simulink model "sedemo_absbrake_can"  (Simulink 7.5)
settings: Solver=ode45  SolverMode=SingleTasking  StartTime=0.0  StopTime=17  MaxStep=inf  RelTol=2e-2  AbsTol=1e-4
PreLoadFcn:
  | sedemo_absdata;
  | BUSCapacity = 50000;
StopFcn:
  | if exist ('logsout')
  | tagName = 'Net';
  | sedemo_absbrakeplots_delay;
  | clear figExt tagName;
  | end
values from neighbouring files (symbols this model uses):
  ctrl = 1    [sedemo_absdata.m]
  g = 32.18    [sedemo_absdata.m]
  I = 5    [sedemo_absdata.m]
  Kf = 1    [sedemo_absdata.m]
  m = 50    [sedemo_absdata.m]
  mu = [0 .4 .8 .97 1.0 .98 .96 .94 .92 .9 .88 .855 .83 .81 .79 .77 .75 .73 .72 .71 .7]    [sedemo_absdata.m]
  PBmax = 1500    [sedemo_absdata.m]
  Rr = 15/12    (= 1.25)    [sedemo_absdata.m]
  slip = (0:.05:1.0)    [sedemo_absdata.m]
  TB = 0.01    [sedemo_absdata.m]
  v0 = 88    [sedemo_absdata.m]
undefined symbols (not defined in the file or in its folder): des_subsystemblock, des_subsysteminport, des_subsystemoutport, des_subsystemsupportblock
libraries: simeventsrouting1 x30, simeventstranslate1 x25, simeventssink1 x21, simeventsserver1 x19, simeventsattributes2 x15, simeventsgates1 x10, simeventsqueue1 x6, simulink x5, simeventsgenerators1 x5, simeventssignalmanage1 x5, simeventstiming1 x3, simeventsinfo x1
(part 1 of 4)
CloseFcn:
  | tagName = 'Net';
  | h = findobj(0, 'Name', 'ABS Speeds', 'Tag', tagName);
  | delete(h);
  | h = findobj(0, 'Name',  'ABS Slip', 'Tag', tagName);
  | delete(h);
  | clear h figExt tagName I PBmax Sd Vs ctrl logsout mu slp v0;
  | clear Kf Rr TB Ww g m slip time BUSCapacity;
  | clear global BUSCapacity;
settings Model: Creator=The MathWorks Inc.  ExtModeTrigMode=oneshot  ExtModeArmWhenConnect=off  ExtModeAutoUpdateStatusClock=off
settings DataIOCC: LimitDataPoints=off  SaveOutput=off  SaveTime=off  TimeSaveName=time
settings OptimizationCC: InlineParams=on  InlineInvariantSignals=on  InitFltsAndDblsToZero=on  EfficientMapNaN2IntZero=off  BufferReusableBoundary=off
settings DebuggingCC: SignalResolutionControl=TryResolveAllWithWarning  SolverPrmCheckMsg=none  MultiTaskDSMMsg=warning  MultiTaskCondExecSysMsg=none  SigSpecEnsureSampleTimeMsg=none  IntegerOverflowMsg=none  BusObjectLabelMismatch=none  StrictBusMsg=None
settings HardwareCC: TargetUnknown=on
settings RTWCC: IncludeERTFirstTime=on
settings SimEventsCC: propMaxDesBlkSimulEvents=10000  propDiagAttribOutput=1  propDiagFcnCallOutput=1  propDiagStatOutput=0

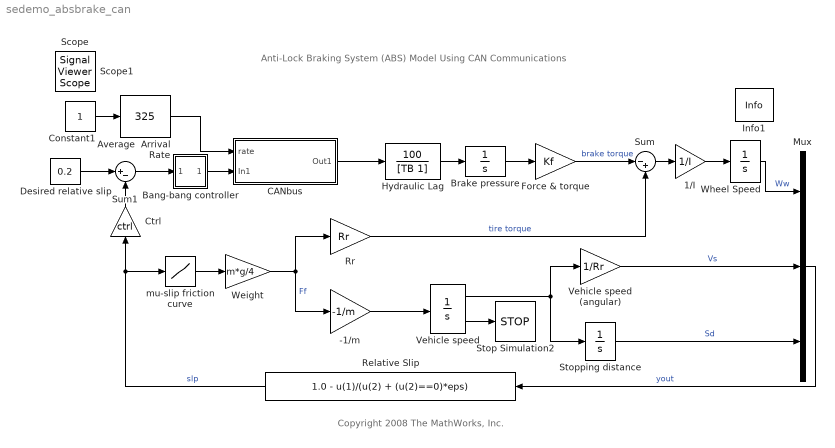
== system sedemo_absbrake_can ==
  note: Anti-Lock Braking System (ABS) Model Using CAN Communications
  note: Copyright 2008 The MathWorks, Inc.
  -1/m : Gain  Gain=-1/m  ParameterDataType=sfix(16)  ParameterScaling=2^0  OutDataType=sfix(16)  OutScaling=2^0  SaturateOnIntegerOverflow=on  OutDataTypeStr=Inherit: Same as input  ParamDataTypeStr=Inherit: Same as input
  1/I : Gain  Gain=1/I  ParameterDataType=sfix(16)  ParameterScaling=2^0  OutDataType=sfix(16)  OutScaling=2^0  SaturateOnIntegerOverflow=on  OutDataTypeStr=Inherit: Same as input  ParamDataTypeStr=Inherit: Same as input
  Average  Arrival Rate : simulink/Math Operations/Slider Gain  SystemSampleTime=-1  low=0  gain=325  high=450
  Bang-bang controller : Subsystem
      mask Type: Sign
      mask Description: y = sign(x)
      mask Help: Sign Function:\n\t\t\ty = 1 if x > 0\n\t\t\ty = 0 if x = 0\n\t\t\ty = -1 if x < 0
      mask Display: plot(-50,-50,50,50,[-50,50],[0,0],[0,0],[-50,50],[-40,0],[-30,-30],[0,40],[30,30])
  Brake pressure : Integrator  LimitOutput=on  UpperSaturationLimit=PBmax  LowerSaturationLimit=0
  CANbus : Subsystem
  Constant1 : Constant  OutDataType=sfix(16)  OutScaling=2^0
  Ctrl : Gain  Gain=ctrl  ParameterDataType=sfix(16)  ParameterScaling=2^0  OutDataType=sfix(16)  OutScaling=2^0  SaturateOnIntegerOverflow=on  OutDataTypeStr=Inherit: Same as input  ParamDataTypeStr=Inherit: Same as input
  Desired relative slip : Constant  Value=0.2  OutDataType=sfix(16)  OutScaling=2^0
  Force & torque : Gain  Gain=Kf  ParameterDataType=sfix(16)  ParameterScaling=2^0  OutDataType=sfix(16)  OutScaling=2^0  SaturateOnIntegerOverflow=on  OutDataTypeStr=Inherit: Same as input  ParamDataTypeStr=Inherit: Same as input
  "Hydraulic Lag " : TransferFcn  Numerator=[100]  Denominator=[TB 1]
  Info1 : simeventsinfo/Info  SystemSampleTime=-1
  Mux : Mux  Inputs=3
  Relative Slip : Fcn  Expr=1.0 - u(1)/(u(2) + (u(2)==0)*eps)
  Rr : Gain  Gain=Rr  ParameterDataType=sfix(16)  ParameterScaling=2^0  OutDataType=sfix(16)  OutScaling=2^0  SaturateOnIntegerOverflow=on  OutDataTypeStr=Inherit: Same as input  ParamDataTypeStr=Inherit: Same as input
  Stop Simulation2 : Stop
  Stopping distance : Integrator  UpperSaturationLimit=1000  LowerSaturationLimit=0
  Sum : Sum  Inputs=|-+  OutDataType=sfix(16)  OutScaling=2^0  SaturateOnIntegerOverflow=on  InputSameDT=on  OutDataTypeStr=Inherit: Same as first input
  Sum1 : Sum  Inputs=|+-  OutDataType=sfix(16)  OutScaling=2^0  SaturateOnIntegerOverflow=on  InputSameDT=on  OutDataTypeStr=Inherit: Same as first input
  Vehicle speed : Integrator  InitialCondition=v0  LimitOutput=on  UpperSaturationLimit=1000  LowerSaturationLimit=0  ShowSaturationPort=on
  Vehicle speed (angular) : Gain  Gain=1/Rr  ParameterDataType=sfix(16)  ParameterScaling=2^0  OutDataType=sfix(16)  OutScaling=2^0  SaturateOnIntegerOverflow=on  OutDataTypeStr=Inherit: Same as input  ParamDataTypeStr=Inherit: Same as input
  Weight : Gain  Gain=m*g/4  ParameterDataType=sfix(16)  ParameterScaling=2^0  OutDataType=sfix(16)  OutScaling=2^0  SaturateOnIntegerOverflow=on  OutDataTypeStr=Inherit: Same as input  ParamDataTypeStr=Inherit: Same as input
  Wheel Speed : Integrator  InitialCondition=v0/Rr  LimitOutput=on  UpperSaturationLimit=1000  LowerSaturationLimit=0
  mu-slip friction curve : Lookup  InputValues=slip  Table=mu  OutDataType=sfix(16)  OutScaling=2^0  SaturateOnIntegerOverflow=on
  Scope : SignalViewerScope  IOType=viewer  RefreshTime=0.035000
      settings: TimeRange=15  YMin=0  YMax=800
  Scope1 : SignalViewerScope  IOType=viewer  RefreshTime=0.035000
      settings: TimeRange=15  YMin=0  YMax=1
  wires:
  Mux/1 -> Relative Slip/1  "yout"
  Vehicle speed (angular)/1 -> Mux/2  "Vs"
  Relative Slip/1 -> mu-slip friction curve/1, Ctrl/1  "slp"
  Stopping distance/1 -> Mux/3  "Sd"
  -1/m/1 -> Vehicle speed/1
  Vehicle speed/2 -> Stop Simulation2/1
  Vehicle speed/1 -> Stopping distance/1, Vehicle speed (angular)/1
  mu-slip friction curve/1 -> Weight/1
  Weight/1 -> -1/m/1, Rr/1  "Ff"
  Ctrl/1 -> Sum1/2
  Desired relative slip/1 -> Sum1/1
  Sum1/1 -> Bang-bang controller/1(in_1)
  Wheel Speed/1 -> Mux/1  "Ww"
  Rr/1 -> Sum/2  "tire torque"
  1/I/1 -> Wheel Speed/1
  Sum/1 -> 1/I/1
  Force & torque/1 -> Sum/1  "brake torque"
  Brake pressure/1 -> Force & torque/1
  "Hydraulic Lag "/1 -> Brake pressure/1
  Constant1/1 -> Average  Arrival Rate/1
  Average  Arrival Rate/1 -> CANbus/1(rate)
  Bang-bang controller/1(out_1) -> CANbus/2(In1)
  CANbus/1(Out1) -> "Hydraulic Lag "/1

== system sedemo_absbrake_can/Bang-bang controller ==
  in_1 : Inport  OutDataType=sfix(16)  OutScaling=2^0
  Constant : Constant  Value=0  OutDataType=sfix(16)  OutScaling=2^0
  Data Type Conversion1 : DataTypeConversion  OutDataTypeMode=double  OutDataType=sfix(16)  OutScaling=2^0  OutDataTypeStr=double  SaturateOnIntegerOverflow=on  RndMeth=Zero
  Data Type Conversion2 : DataTypeConversion  OutDataTypeMode=double  OutDataType=sfix(16)  OutScaling=2^0  OutDataTypeStr=double  SaturateOnIntegerOverflow=on  RndMeth=Zero
  Relational Operator : RelationalOperator  Operator=>  InputSameDT=on
  Relational Operator1 : RelationalOperator  Operator=<  InputSameDT=on
  Sum : Sum  Inputs=+-  OutDataType=sfix(16)  OutScaling=2^0  SaturateOnIntegerOverflow=on  InputSameDT=on  OutDataTypeStr=Inherit: Same as first input
  out_1 : Outport  OutDataType=sfix(16)  OutScaling=2^0  InitialOutput=0
  wires:
  Data Type Conversion2/1 -> Sum/2
  Data Type Conversion1/1 -> Sum/1
  Sum/1 -> out_1/1
  Relational Operator/1 -> Data Type Conversion1/1
  Relational Operator1/1 -> Data Type Conversion2/1
  Constant/1 -> Relational Operator/2, Relational Operator1/2
  in_1/1 -> Relational Operator1/1, Relational Operator/1

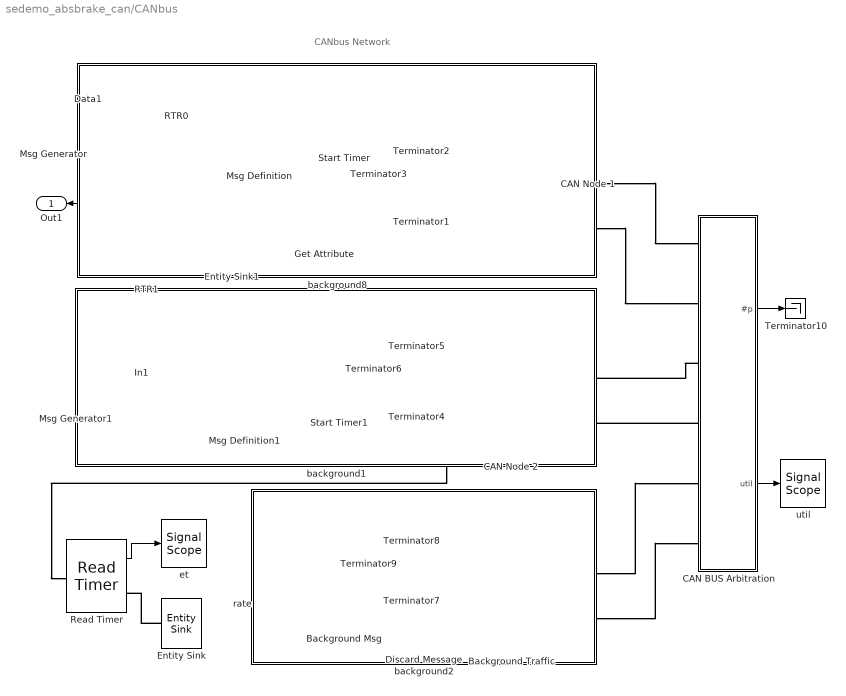
== system sedemo_absbrake_can/CANbus ==
  note: CANbus Network
  rate : Inport  OutDataType=sfix(16)  OutScaling=2^0
  In1 : Inport  Port=2  OutDataType=sfix(16)  OutScaling=2^0
  Background Msg : Subsystem
  Background Traffic : Subsystem  mask(Background Traffic){IDRange=[0:9], IDSubscription=[zeros(1,10)]}
      mask prompts: IDRange "Message ID"; IDSubscription "Subscription (0-no, 1-yes)"
      mask help: Transmits and receives messages to and from multiple nodes over the CANbus to represent background traffic on the CANbus.
  CAN BUS Arbitration : Subsystem  mask{Capacity=50000, LossRate=0.001}
      mask prompts: Capacity "Channel capacity(bit/s)"; LossRate "Loss probability(0-1)"
      mask init:
      | global BUSCapacity;
      | BUSCapacity = Capacity;
  CAN Node 1 : Subsystem  mask(CAN Node){IDRange=[0:9], IDSubscription=[0,0,0,1,0,0,0,0,0,0]}
      mask prompts: IDRange "Message ID"; IDSubscription "Subscription (0-no, 1-yes)"
      mask help: CAN Node transmits and receives messages over the CANbus.
  CAN Node 2 : Subsystem  mask(CAN Node){IDRange=[0:9], IDSubscription=[0,0,1,0,0,0,0,0,0,0]}
      mask prompts: IDRange "Message ID"; IDSubscription "Subscription (0-no, 1-yes)"
      mask help: CAN Node transmits and receives messages over the CANbus.
  Data1 : simulink/Sources/Ramp  SystemSampleTime=-1  slope=1  start=0  X0=0
  Discard Message : simeventssink1/Entity Sink  Priority=1  SystemSampleTime=-1  AvailableForArrivals=on  StatNumberArrived=Off
  Entity Sink : simeventssink1/Entity Sink  Priority=1  SystemSampleTime=-1  AvailableForArrivals=on  StatNumberArrived=Off
  Entity Sink1 : simeventssink1/Entity Sink  Priority=1  SystemSampleTime=-1  AvailableForArrivals=on  StatNumberArrived=Off
  Get Attribute : simeventsattributes2/Get Attribute  Priority=1  DialogController=des_ddg_create  DialogControllerArgs=DataTag206  SystemSampleTime=-1  AttributeName=Data  AttributeMissing=Error  AttributeDefaultValue=1  AttributeSendTiming=After entity departure  AttributeTreatAsVector=1  StatNumberDeparted=Off  EvaluatedDefaultAttributeValue={[]}
  Msg Definition : Subsystem  mask{MsgID=2, MsgSize=8}
      mask prompts: MsgID "CAN identifier (ID)"; MsgSize "Data size (0-8 bytes)"
      settings: AttributesFormatString=(ID = %<MsgID>)
  Msg Definition1 : Subsystem  mask{MsgID=3, MsgSize=8}
      mask prompts: MsgID "CAN identifier (ID)"; MsgSize "Data size (0-8 bytes)"
      settings: AttributesFormatString=(ID = %<MsgID>)
  Msg Generator : simeventsgenerators1/Entity Generators/Time-Based Entity Generator  Priority=1  DialogController=des_ddg_create  DialogControllerArgs=DataTag212  SystemSampleTime=-1  GenerateEntitiesUpon=Intergeneration time from dialog  Distribution=Constant  Minimum=0  Maximum=1  Mean=0.05  InitialSeed=568654  Period=0.333  PriorityEntityGeneration=300  GenerateEntityAtSimulationStart=off  ResponseWhenBlocked=Pause generation  ResponseWhenUnblocked=Immediate restart  EntityType=Standard  StatNumberDeparted=Off  StatPendingEntity=Off  StatAverageIntergenerationTime=Off
  Msg Generator1 : simeventsgenerators1/Entity Generators/Time-Based Entity Generator  Priority=1  DialogController=des_ddg_create  DialogControllerArgs=DataTag214  SystemSampleTime=-1  GenerateEntitiesUpon=Intergeneration time from dialog  Distribution=Constant  Minimum=0  Maximum=1  Mean=0.05  InitialSeed=5363461  Period=0.01  PriorityEntityGeneration=300  GenerateEntityAtSimulationStart=off  ResponseWhenBlocked=Pause generation  ResponseWhenUnblocked=Immediate restart  EntityType=Standard  StatNumberDeparted=Off  StatPendingEntity=Off  StatAverageIntergenerationTime=Off
  RTR0 : Constant  Value=0  OutDataType=sfix(16)  OutScaling=2^0
  RTR1 : Constant  Value=0  OutDataType=sfix(16)  OutScaling=2^0
  Read Timer : simeventstiming1/Read Timer  Priority=0  SystemSampleTime=-1  TimerTag=T1  TimerModeOption=Error  TimerStop=off  StatNumberDeparted=Off  StatTimerNumberDeparted=Off  StatTimeElapsed=On  StatAverageTimeElapsed=Off
  Start Timer : simeventstiming1/Start Timer  Priority=0  SystemSampleTime=-1  TimerTag=T1  TimerStartedOption=Warn and continue  StatNumberDeparted=Off
  Start Timer1 : simeventstiming1/Start Timer  Priority=0  SystemSampleTime=-1  TimerTag=T1  TimerStartedOption=Warn and continue  StatNumberDeparted=Off
  Terminator{1..10} (10 alike) : Terminator
  background1 : Subsystem
      mask Display: disp('')
  background2 : Subsystem
      mask Display: disp('')
  background8 : Subsystem
      mask Display: disp('')
  et : simeventssink1/Signal Scope  Priority=1  SystemSampleTime=-1  PlotType=Stair  InputType=Signal  NumInputs=1  AttributeNameY=Count  XInputOptionSignal=Event time  XInputOptionEntity=Event time  AttributeNameX=Count  EnableEntityOutport=on  XMin=0  XMax=18  XLimitExceededOption=Stretch axis limits  YLimitExceededOption=Stretch axis limits  AxisGrid=on  AxisLegend=off  LineDisables=""  LineColors=b  LineStyles=-  LineMarkers=None  OpenScopeAtSimStart=on  Title=Message Delivery Delay  YLabel=Delay  XLabel=Time  FigurePosition=[461 438 307 230]  AxisZoom=off  DataStoreOption=Unlimited  DataPointsLimit=10000  StatNumberArrived=Off  ShowCountPlotted=off  ShowToolbar=off
      settings: YMin=0  YMax=0.005
  util : simeventssink1/Signal Scope  Priority=1  SystemSampleTime=-1  PlotType=Stair  InputType=Signal  NumInputs=1  AttributeNameY=Count  XInputOptionSignal=Event time  XInputOptionEntity=Event time  AttributeNameX=Count  EnableEntityOutport=on  XMin=0  XMax=18  XLimitExceededOption=Stretch axis limits  YLimitExceededOption=Stretch axis limits  AxisGrid=on  AxisLegend=off  LineDisables=""  LineColors=b  LineStyles=-  LineMarkers=None  OpenScopeAtSimStart=on  Title=CANbus Network Utilization  YLabel=Utilization  XLabel=Time  FigurePosition=[51 437 307 230]  AxisZoom=off  DataStoreOption=Unlimited  DataPointsLimit=10000  StatNumberArrived=Off  ShowCountPlotted=off  ShowToolbar=off
      settings: YMin=0  YMax=1
  Out1 : Outport  OutDataType=sfix(16)  OutScaling=2^0
  wires:
  Get Attribute/1 -> Out1/1
  rate/1 -> Background Msg/1(rate)
  CAN BUS Arbitration/1(#p) -> Terminator10/1
  CAN BUS Arbitration/2(util) -> util/1
  Background Traffic/4(#Tx) -> Terminator7/1
  Background Traffic/3(#OF) -> Terminator9/1
  Background Traffic/1(#Rx) -> Terminator8/1
  Background Traffic/2(#Bx) -> Background Traffic/1(Idx)
  Read Timer/1 -> et/1
  CAN Node 2/4(#Tx) -> Terminator4/1
  CAN Node 2/3(#OF) -> Terminator6/1
  CAN Node 2/1(#Rx) -> Terminator5/1
  RTR1/1 -> Msg Definition1/1(RTR)
  In1/1 -> Msg Definition1/2(Data)
  CAN Node 2/2(#Bx) -> CAN Node 2/1(Idx)
  CAN Node 1/4(#Tx) -> Terminator1/1
  CAN Node 1/3(#OF) -> Terminator3/1
  CAN Node 1/1(#Rx) -> Terminator2/1
  RTR0/1 -> Msg Definition/1(RTR)
  Data1/1 -> Msg Definition/2(Data)
  CAN Node 1/2(#Bx) -> CAN Node 1/1(Idx)
  connections:
  Entity Sink1/LConn1 -- Get Attribute/RConn1
  Get Attribute/LConn1 -- CAN Node 1/RConn2
  Background Msg/RConn1 -- Background Traffic/RConn1
  CAN Node 1/LConn2 -- CAN BUS Arbitration/LConn2
  CAN Node 1/LConn1 -- CAN BUS Arbitration/LConn1
  Entity Sink/LConn1 -- Read Timer/RConn1
  Msg Generator/RConn1 -- Msg Definition/LConn1
  Start Timer1/RConn1 -- CAN Node 2/RConn1
  Background Traffic/LConn2 -- CAN BUS Arbitration/LConn6
  Msg Definition/RConn1 -- Start Timer/LConn1
  Msg Generator1/RConn1 -- Msg Definition1/LConn1
  Msg Definition1/RConn1 -- Start Timer1/LConn1
  Start Timer/RConn1 -- CAN Node 1/RConn1
  CAN BUS Arbitration/LConn3 -- CAN Node 2/LConn1
  Background Traffic/LConn1 -- CAN BUS Arbitration/LConn5
  CAN Node 2/RConn2 -- Read Timer/LConn1
  CAN BUS Arbitration/LConn4 -- CAN Node 2/LConn2
  Discard Message/LConn1 -- Background Traffic/RConn2

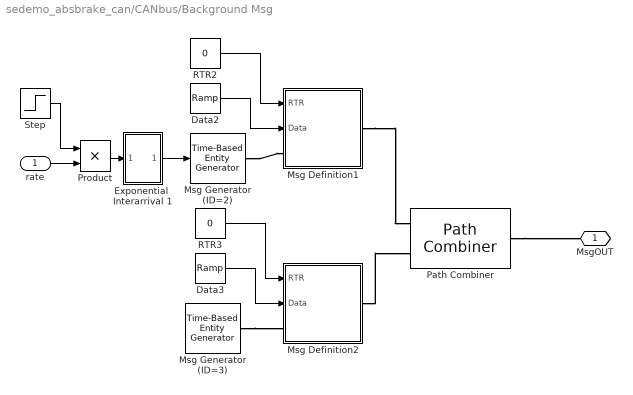
== system sedemo_absbrake_can/CANbus/Background Msg ==
  rate : Inport  OutDataType=sfix(16)  OutScaling=2^0
  Data2 : simulink/Sources/Ramp  SystemSampleTime=-1  slope=1  start=0  X0=0
  Data3 : simulink/Sources/Ramp  SystemSampleTime=-1  slope=1  start=0  X0=0
  Exponential  Interarrival 1 : Subsystem  mask(Exponential Random Number Generator){seed=0546269209}
      mask prompts: seed "Initial seed"
      mask help: Generate random numbers with an exponential distribution. User can specify the rate and the initial seed.
      mask Display: plot([0.4 .13 .38 .26 .71 .44 .6 .15 .22 .5 .55 .6 .4]);
  Msg Definition1 : Subsystem  mask{MsgID=0, MsgSize=8}
      mask prompts: MsgID "CAN identifier (ID)"; MsgSize "Data size (0-8 bytes)"
      settings: AttributesFormatString=(ID = %<MsgID>)
  Msg Definition2 : Subsystem  mask{MsgID=1, MsgSize=8}
      mask prompts: MsgID "CAN identifier (ID)"; MsgSize "Data size (0-8 bytes)"
      settings: AttributesFormatString=(ID = %<MsgID>)
  Msg Generator (ID=2) : simeventsgenerators1/Entity Generators/Time-Based Entity Generator  Priority=1  DialogController=des_ddg_create  DialogControllerArgs=DataTag5  SystemSampleTime=-1  GenerateEntitiesUpon=Intergeneration time from port t  Distribution=Exponential  Minimum=0  Maximum=1  Mean=0.02  InitialSeed=67457  Period=0.05  PriorityEntityGeneration=300  GenerateEntityAtSimulationStart=off  ResponseWhenBlocked=Pause generation  ResponseWhenUnblocked=Immediate restart  EntityType=Standard  StatNumberDeparted=Off  StatPendingEntity=Off  StatAverageIntergenerationTime=Off
  Msg Generator (ID=3) : simeventsgenerators1/Entity Generators/Time-Based Entity Generator  Priority=1  DialogController=des_ddg_create  DialogControllerArgs=DataTag7  SystemSampleTime=-1  GenerateEntitiesUpon=Intergeneration time from dialog  Distribution=Constant  Minimum=.04  Maximum=.1  Mean=0.08  InitialSeed=3767  Period=inf  PriorityEntityGeneration=300  GenerateEntityAtSimulationStart=off  ResponseWhenBlocked=Pause generation  ResponseWhenUnblocked=Immediate restart  EntityType=Standard  StatNumberDeparted=Off  StatPendingEntity=Off  StatAverageIntergenerationTime=Off
  Path Combiner : simeventsrouting1/Path Combiner  Priority=1  SystemSampleTime=-1  NumberInputPorts=2  InputPortPrecedence=IN1 port  InitialSeed=45675  SpecifyEventPriority=off  PriorityPathCombinerPortPrecedenceSelection=4100  StatNumberDeparted=Off  StatLastArrivalPort=Off  EvaluatedNumPorts=2
  Product : Product  OutDataType=sfix(16)  OutScaling=2^0  RndMeth=Zero
  RTR2 : Constant  Value=0  OutDataType=sfix(16)  OutScaling=2^0
  RTR3 : Constant  Value=0  OutDataType=sfix(16)  OutScaling=2^0
  Step : Step  Time=6  Before=.01  SampleTime=0
  MsgOUT : PMIOPort  Port=1  Side=Right
  wires:
  rate/1 -> Product/2
  Product/1 -> Exponential  Interarrival 1/1(rate)
  Step/1 -> Product/1
  Exponential  Interarrival 1/1(Out1) -> Msg Generator (ID=2)/1
  RTR3/1 -> Msg Definition2/1(RTR)
  Data3/1 -> Msg Definition2/2(Data)
  RTR2/1 -> Msg Definition1/1(RTR)
  Data2/1 -> Msg Definition1/2(Data)
  connections:
  Msg Definition1/RConn1 -- Path Combiner/LConn1
  Msg Definition2/RConn1 -- Path Combiner/LConn2
  Path Combiner/RConn1 -- MsgOUT/RConn1
  Msg Generator (ID=3)/RConn1 -- Msg Definition2/LConn1
  Msg Generator (ID=2)/RConn1 -- Msg Definition1/LConn1

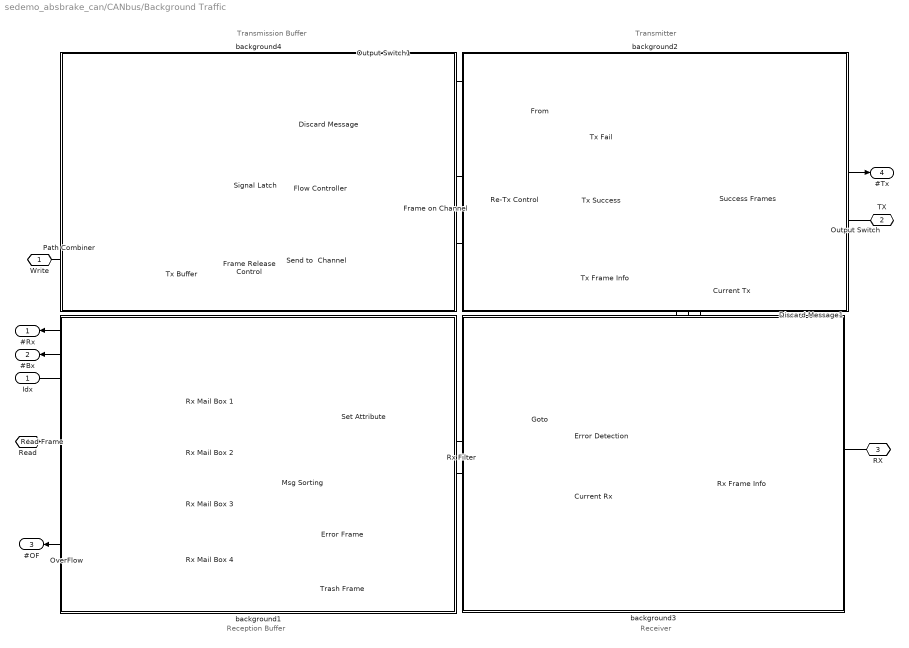
== system sedemo_absbrake_can/CANbus/Background Traffic ==
  note: Reception Buffer
  note: Transmission Buffer
  note: Transmitter
  note: Receiver
  Idx : Inport  OutDataType=sfix(16)  OutScaling=2^0
  Current Rx : simeventsserver1/Single Server  Priority=1  SystemSampleTime=-1  ServiceTimeFrom=Dialog  ServiceTime=0  AttributeName=ServiceTime  PriorityServiceCompletion=2400  PermitPreemption=off  SortingAttributeName=ID  SortingDirection=Ascending  WriteToAttribute=off  ResidualAttributeName=ResidualServiceTime  CreateAttribute=on  EnableTOPort=off  StatNumberDeparted=Off  StatNumberInBlock=Off  StatNumberPreempted=Off  StatPendingEntity=Off  StatAverageWait=Off  StatUtilization=Off  StatNumberTimedout=Off
  Current Tx : simeventsserver1/Single Server  Priority=1  SystemSampleTime=-1  ServiceTimeFrom=Dialog  ServiceTime=0  AttributeName=ServiceTime  PriorityServiceCompletion=2400  PermitPreemption=off  SortingAttributeName=ID  SortingDirection=Ascending  WriteToAttribute=off  ResidualAttributeName=ResidualServiceTime  CreateAttribute=on  EnableTOPort=off  StatNumberDeparted=Off  StatNumberInBlock=Off  StatNumberPreempted=Off  StatPendingEntity=Off  StatAverageWait=Off  StatUtilization=Off  StatNumberTimedout=Off
  Discard Message : simeventssink1/Entity Sink  Priority=1  SystemSampleTime=-1  AvailableForArrivals=on  StatNumberArrived=Off
  Discard Message1 : simeventssink1/Entity Sink  Priority=1  SystemSampleTime=-1  AvailableForArrivals=on  StatNumberArrived=Off
  Error Detection : Subsystem  LoadFcn=des_subsystemblock(gcb, 'load');  InitFcn=des_subsystemblock(gcb, 'init');  StartFcn=des_subsystemblock(gcb, 'start');  StopFcn=des_subsystemblock(gcb, 'stop');
      settings: CopyFcn=des_subsystemblock(gcb, 'copy');  DeleteFcn=des_subsystemblock(gcb, 'delete');  UndoDeleteFcn=des_subsystemblock(gcb, 'undodelete');  ModelCloseFcn=des_subsystemblock(gcb, 'modelclose');  PreSaveFcn=des_subsystemblock(gcb, 'presave');  NameChangeFcn=des_subsystemblock(gcb, 'namechange');  ParentCloseFcn=des_subsystemblock(gcb, 'parentclose');  ErrorFcn=des_subsystemerror
  Error Frame : simeventssink1/Entity Sink  Priority=1  SystemSampleTime=-1  AvailableForArrivals=on  StatNumberArrived=Off
  Flow Controller : Subsystem  LoadFcn=des_subsystemblock(gcb, 'load');  InitFcn=des_subsystemblock(gcb, 'init');  StartFcn=des_subsystemblock(gcb, 'start');  StopFcn=des_subsystemblock(gcb, 'stop');
      settings: CopyFcn=des_subsystemblock(gcb, 'copy');  DeleteFcn=des_subsystemblock(gcb, 'delete');  UndoDeleteFcn=des_subsystemblock(gcb, 'undodelete');  ModelCloseFcn=des_subsystemblock(gcb, 'modelclose');  PreSaveFcn=des_subsystemblock(gcb, 'presave');  NameChangeFcn=des_subsystemblock(gcb, 'namechange');  ParentCloseFcn=des_subsystemblock(gcb, 'parentclose');  ErrorFcn=des_subsystemerror
  Frame Release Control : simeventsgates1/Enabled Gate  Priority=1  SystemSampleTime=-1  SpecifyEventPriority=on  PriorityGateEnableOpenClose=2300  StatNumberDeparted=Off
  Frame on Channel : simeventsqueue1/FIFO Queue  Priority=1  SystemSampleTime=-1  Capacity=2  EnableTOPort=off  StatNumberDeparted=Off  StatNumberInBlock=On  StatPendingEntity=Off  StatAverageWait=Off  StatAverageQueueLength=Off  StatNumberTimedout=Off
  Msg Sorting : simeventsrouting1/Output Switch  Priority=1  SystemSampleTime=-1  NumberOutputPorts=4  SwitchingCriterion=Round robin  InitialSeed=34567  AttributeName=Attribute1  InitialConditionsOpt=off  InitialConditions=1  EntityBufferOpt=off  SpecifyEventPriority=off  PriorityOutputSwitchSelectPort=4100  TimeoutPortOpt=off  StatNumberDeparted=On  StatNumberTimedOut=Off  StatPendingEntity=Off  StatLastDeparturePort=On  EvaluatedNumPorts=4
  Output Switch : simeventsrouting1/Output Switch  Priority=1  SystemSampleTime=-1  NumberOutputPorts=2  SwitchingCriterion=First port that is not blocked  InitialSeed=34567  AttributeName=Attribute1  InitialConditionsOpt=off  InitialConditions=1  EntityBufferOpt=off  SpecifyEventPriority=off  PriorityOutputSwitchSelectPort=4100  TimeoutPortOpt=off  StatNumberDeparted=Off  StatNumberTimedOut=Off  StatPendingEntity=Off  StatLastDeparturePort=Off  EvaluatedNumPorts=2
  Output Switch1 : simeventsrouting1/Output Switch  Priority=1  SystemSampleTime=-1  NumberOutputPorts=2  SwitchingCriterion=First port that is not blocked  InitialSeed=34567  AttributeName=Attribute1  InitialConditionsOpt=off  InitialConditions=1  EntityBufferOpt=off  SpecifyEventPriority=off  PriorityOutputSwitchSelectPort=4100  TimeoutPortOpt=off  StatNumberDeparted=Off  StatNumberTimedOut=Off  StatPendingEntity=Off  StatLastDeparturePort=Off  EvaluatedNumPorts=2
  OverFlow : simeventsrouting1/Path Combiner  Priority=1  SystemSampleTime=-1  NumberInputPorts=4  InputPortPrecedence=IN1 port  InitialSeed=45675  SpecifyEventPriority=off  PriorityPathCombinerPortPrecedenceSelection=4100  StatNumberDeparted=On  StatLastArrivalPort=Off  EvaluatedNumPorts=4
  Path Combiner : simeventsrouting1/Path Combiner  Priority=1  SystemSampleTime=-1  NumberInputPorts=2  InputPortPrecedence=IN1 port  InitialSeed=45675  SpecifyEventPriority=off  PriorityPathCombinerPortPrecedenceSelection=4100  StatNumberDeparted=Off  StatLastArrivalPort=Off  EvaluatedNumPorts=2
  Re-Tx Control : simeventsrouting1/Output Switch  Priority=1  SystemSampleTime=-1  NumberOutputPorts=2  SwitchingCriterion=First port that is not blocked  InitialSeed=34567  AttributeName=Attribute1  InitialConditionsOpt=off  InitialConditions=1  EntityBufferOpt=off  SpecifyEventPriority=off  PriorityOutputSwitchSelectPort=4100  TimeoutPortOpt=off  StatNumberDeparted=Off  StatNumberTimedOut=Off  StatPendingEntity=Off  StatLastDeparturePort=Off  EvaluatedNumPorts=2
  Read Frame : simeventsrouting1/Input Switch  Priority=1  SystemSampleTime=-1  NumberInputPorts=4  SwitchingCriterion=From signal port p  InitialSeed=23453  SpecifyEventPriority=off  PriorityInputSwitchSelectPort=4000  StatNumberDeparted=Off  StatLastArrivalPort=Off  EvaluatedNumPorts=4
  Rx Filter : simeventsrouting1/Output Switch  Priority=1  SystemSampleTime=-1  NumberOutputPorts=3  SwitchingCriterion=From signal port p  InitialSeed=34567  AttributeName=Attribute1  InitialConditionsOpt=off  InitialConditions=1  EntityBufferOpt=off  SpecifyEventPriority=off  PriorityOutputSwitchSelectPort=4100  TimeoutPortOpt=off  StatNumberDeparted=On  StatNumberTimedOut=Off  StatPendingEntity=Off  StatLastDeparturePort=Off  EvaluatedNumPorts=3
  Rx Frame Info : simeventsattributes2/Get Attribute  Priority=1  DialogController=des_ddg_create  DialogControllerArgs=DataTag52  SystemSampleTime=-1  AttributeName=ID|RndLoss|RTR|Data  AttributeMissing=Error|Error|Error|Error  AttributeDefaultValue=1|1|1|1  AttributeSendTiming=After entity departure|After entity departure|After entity departure|After entity departure  AttributeTreatAsVector=1|1|1|1  StatNumberDeparted=Off  EvaluatedDefaultAttributeValue={[];[];[];[]}
  Rx Mail Box {1..4} (4 alike) : simeventsserver1/Single Server  Priority=1  SystemSampleTime=-1  ServiceTimeFrom=Dialog  ServiceTime=0  AttributeName=ServiceTime  PriorityServiceCompletion=2400  PermitPreemption=on  SortingAttributeName=time  SortingDirection=Descending  WriteToAttribute=off  ResidualAttributeName=ResidualServiceTime  CreateAttribute=on  EnableTOPort=off  StatNumberDeparted=Off  StatNumberInBlock=Off  StatNumberPreempted=Off  StatPendingEntity=Off  StatAverageWait=Off  StatUtilization=Off  StatNumberTimedout=Off
  Send to  Channel : simeventsrouting1/Replicate  Priority=1  SystemSampleTime=-1  NumberOutputPorts=2  ReplicateEntityWhen=All entity output ports are not blocked  OutputPortPrecedence=OUT1 port  InitialSeed=56789  ActionUponBlocking=Discard entity  StatNumberArrived=Off  StatNumberDeparted=Off  EvaluatedNumPorts=2
  Set Attribute : simeventsattributes2/Set Attribute  Priority=1  DialogController=des_ddg_create  DialogControllerArgs=DataTag59  SystemSampleTime=-1  AttributeFrom=Signal port  AttributeName=time  AttributeTreatAsVector=1  AttributeValue=1  AttributeCreate=on  StatNumberDeparted=Off  EvaluatedAttributeValue={[]}
  Signal Latch : simeventssignalmanage1/Signal Latch  Priority=1  SystemSampleTime=-1  InitialMemoryValue=1  WriteMemoryUpon=Sample time hit from port wts  MemoryWriteEdgeOption=Either  SpecifyWriteEventPriority=on  PriorityMemoryWrite=2200  ReadMemoryUpon=Write to memory event  MemoryReadEdgeOption=Falling  SpecifyReadEventPriority=on  PriorityMemoryRead=7000  ReportMemoryState=off  ReportMemoryUponWrite=off  ReportMemoryUponRead=on
  Success Frames : simeventssink1/Entity Sink  Priority=1  SystemSampleTime=-1  AvailableForArrivals=on  StatNumberArrived=On
  Trash Frame : simeventssink1/Entity Sink  Priority=1  SystemSampleTime=-1  AvailableForArrivals=on  StatNumberArrived=Off
  Tx Buffer : simeventsqueue1/Priority Queue  Priority=1  SystemSampleTime=-1  Capacity=15  SortingAttributeName=ID  SortingDirection=Ascending  EnableTOPort=off  StatNumberDeparted=Off  StatNumberInBlock=Off  StatPendingEntity=Off  StatAverageWait=Off  StatAverageQueueLength=Off  StatNumberTimedout=Off
  Tx Fail : simeventsgates1/Release Gate  Priority=1  SystemSampleTime=-1  OpenGateUpon=Change in signal from port vc  SignalEdgeOption=Falling  SpecifyEventPriority=on  PriorityGateRelease=2000  StatNumberDeparted=Off
  Tx Frame Info : simeventsattributes2/Get Attribute  Priority=1  DialogController=des_ddg_create  DialogControllerArgs=DataTag66  SystemSampleTime=-1  AttributeName=ID|RTR|Data  AttributeMissing=Error|Error|Error  AttributeDefaultValue=1|1|1  AttributeSendTiming=After entity departure|After entity departure|After entity departure  AttributeTreatAsVector=1|1|1  StatNumberDeparted=Off  EvaluatedDefaultAttributeValue={[];[];[]}
  Tx Success : simeventsgates1/Release Gate  Priority=1  SystemSampleTime=-1  OpenGateUpon=Change in signal from port vc  SignalEdgeOption=Rising  SpecifyEventPriority=on  PriorityGateRelease=2000  StatNumberDeparted=Off
  background1 : Subsystem
      mask Display: disp('')
  background2 : Subsystem
      mask Display: disp('')
  background3 : Subsystem
      mask Display: disp('')
  background4 : Subsystem
      mask Display: disp('')
  Write : PMIOPort  Port=1  Side=Right
  TX : PMIOPort  Port=2  Side=Left
  RX : PMIOPort  Port=3  Side=Left
  Read : PMIOPort  Port=4  Side=Right
  #Rx : Outport  OutDataType=sfix(16)  OutScaling=2^0
  #Bx : Outport  Port=2  OutDataType=sfix(16)  OutScaling=2^0
  #OF : Outport  Port=3  OutDataType=sfix(16)  OutScaling=2^0
  #Tx : Outport  Port=4  OutDataType=sfix(16)  OutScaling=2^0
  wires:
  Success Frames/1 -> #Tx/1
  Msg Sorting/1 -> #Rx/1
  OverFlow/1 -> #OF/1
  Msg Sorting/2 -> #Bx/1
  Idx/1 -> Read Frame/1
  Signal Latch/1 -> Frame Release Control/1
  Frame on Channel/1 -> Flow Controller/1(busy)
  Rx Filter/1 -> Set Attribute/1
  Rx Frame Info/1 -> Error Detection/1(Rx_ID)
  Rx Frame Info/2 -> Error Detection/2(Loss)
  Tx Frame Info/3 -> Error Detection/7(Tx_Data)
  Tx Frame Info/2 -> Error Detection/6(Tx_RTR)
  Tx Frame Info/1 -> Error Detection/5(Tx_ID)
  Rx Frame Info/3 -> Error Detection/3(Rx_RTR)
  Rx Frame Info/4 -> Error Detection/4(Rx_Data)
  Error Detection/1(Idx) -> Rx Filter/1
  Error Detection/2(ACK) -> [Ack]
  [Ack] -> Tx Fail/1, Tx Success/1
  Flow Controller/1(en) -> Signal Latch/1, Signal Latch/2
  connections:
  Read Frame/RConn1 -- Read/RConn1
  Msg Sorting/RConn4 -- Rx Mail Box 4/LConn1
  Msg Sorting/RConn3 -- Rx Mail Box 3/LConn1
  Msg Sorting/RConn2 -- Rx Mail Box 2/LConn1
  Msg Sorting/RConn1 -- Rx Mail Box 1/LConn1
  Rx Filter/RConn2 -- Error Frame/LConn1
  Current Rx/RConn1 -- Rx Filter/LConn1
  Frame on Channel/RConn1 -- Re-Tx Control/LConn1
  Re-Tx Control/RConn2 -- Tx Success/LConn1
  Re-Tx Control/RConn1 -- Tx Fail/LConn1
  Tx Buffer/RConn1 -- Frame Release Control/LConn1
  Frame Release Control/RConn1 -- Send to  Channel/LConn1
  Path Combiner/RConn1 -- Tx Buffer/LConn1
  Write/RConn1 -- Path Combiner/LConn2
  Tx Success/RConn1 -- Success Frames/LConn1
  Rx Filter/RConn3 -- Trash Frame/LConn1
  Rx Filter/RConn1 -- Set Attribute/LConn1
  Set Attribute/RConn1 -- Msg Sorting/LConn1
  Output Switch/RConn1 -- TX/RConn1
  Tx Fail/RConn1 -- Output Switch1/LConn1
  Output Switch1/RConn1 -- Path Combiner/LConn1
  Rx Frame Info/RConn1 -- Current Rx/LConn1
  Rx Mail Box 4/RConn2 -- OverFlow/LConn4
  Rx Mail Box 3/RConn2 -- OverFlow/LConn3
  Rx Mail Box 2/RConn2 -- OverFlow/LConn2
  Rx Mail Box 1/RConn2 -- OverFlow/LConn1
  Rx Mail Box 1/RConn1 -- Read Frame/LConn1
  Rx Mail Box 2/RConn1 -- Read Frame/LConn2
  Rx Mail Box 3/RConn1 -- Read Frame/LConn3
  Rx Mail Box 4/RConn1 -- Read Frame/LConn4
  RX/RConn1 -- Rx Frame Info/LConn1
  Send to  Channel/RConn2 -- Tx Frame Info/LConn1
  Send to  Channel/RConn1 -- Frame on Channel/LConn1
  Current Tx/RConn1 -- Output Switch/LConn1
  Tx Frame Info/RConn1 -- Current Tx/LConn1
  Discard Message/LConn1 -- Output Switch1/RConn2
  Discard Message1/LConn1 -- Output Switch/RConn2

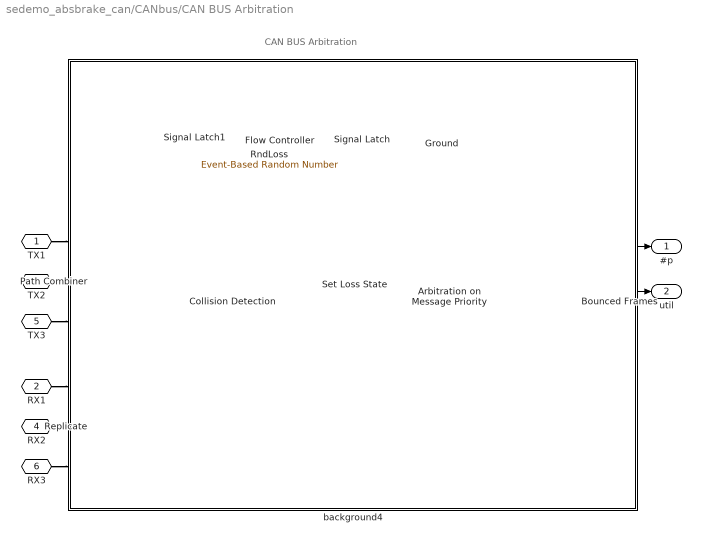
== system sedemo_absbrake_can/CANbus/CAN BUS Arbitration ==
  note: CAN BUS Arbitration
  Arbitration on Message Priority : simeventsserver1/Single Server  Priority=1  SystemSampleTime=-1  ServiceTimeFrom=Attribute  ServiceTime=1  AttributeName=CommDelay  PriorityServiceCompletion=8000  PermitPreemption=on  SortingAttributeName=ID  SortingDirection=Ascending  WriteToAttribute=off  ResidualAttributeName=ResidualServiceTime  CreateAttribute=on  EnableTOPort=off  StatNumberDeparted=Off  StatNumberInBlock=On  StatNumberPreempted=On  StatPendingEntity=Off  StatAverageWait=Off  StatUtilization=On  StatNumberTimedout=Off
  Bounced Frames : simeventssink1/Entity Sink  Priority=1  SystemSampleTime=-1  AvailableForArrivals=on  StatNumberArrived=Off
  Collision Detection : simeventsgates1/Enabled Gate  Priority=1  SystemSampleTime=-1  SpecifyEventPriority=on  PriorityGateEnableOpenClose=200  StatNumberDeparted=Off
  Flow Controller : Subsystem  LoadFcn=des_subsystemblock(gcb, 'load');  InitFcn=des_subsystemblock(gcb, 'init');  StartFcn=des_subsystemblock(gcb, 'start');  StopFcn=des_subsystemblock(gcb, 'stop');
      settings: CopyFcn=des_subsystemblock(gcb, 'copy');  DeleteFcn=des_subsystemblock(gcb, 'delete');  UndoDeleteFcn=des_subsystemblock(gcb, 'undodelete');  ModelCloseFcn=des_subsystemblock(gcb, 'modelclose');  PreSaveFcn=des_subsystemblock(gcb, 'presave');  NameChangeFcn=des_subsystemblock(gcb, 'namechange');  ParentCloseFcn=des_subsystemblock(gcb, 'parentclose');  ErrorFcn=des_subsystemerror
  Ground : Ground
  Path Combiner : simeventsrouting1/Path Combiner  Priority=1  SystemSampleTime=-1  NumberInputPorts=3  InputPortPrecedence=IN1 port  InitialSeed=45675  SpecifyEventPriority=off  PriorityPathCombinerPortPrecedenceSelection=4100  StatNumberDeparted=Off  StatLastArrivalPort=Off  EvaluatedNumPorts=3
  Replicate : simeventsrouting1/Replicate  Priority=1  SystemSampleTime=-1  NumberOutputPorts=3  ReplicateEntityWhen=Any entity output port is not blocked  OutputPortPrecedence=OUT1 port  InitialSeed=56789  ActionUponBlocking=Discard entity  StatNumberArrived=Off  StatNumberDeparted=Off  EvaluatedNumPorts=3
  RndLoss : simeventsgenerators1/Signal Generators/Event-Based Random Number  SystemSampleTime=-1  distribution=Bernoulli  meanExp=1  minUnif=0  maxUnif=1  pOneBern=LossRate  pSuccessBino=0.5  numTrialBino=1  meanNorm=0  stdNorm=1  minTri=1  maxTri=3  modeTri=2  thresholdLogn=0  scaleLogn=1  shapeLogn=1  pSuccessGeo=0.5  meanPoiss=1  thresholdLogl=0  scaleLogl=1  thresholdGam=0  scaleGam=1  shapeGam=1  minBeta=0  maxBeta=1  shape1Beta=1  shape2Beta=1  minUnid=0  maxUnid=1  numValueUnid=2  thresholdWbl=0  scaleWbl=1  shapeWbl=1  valueVecCont=[0 1]  cdfVecCont=[0 1]  valueVecDisc=[0 1]  probVecDisc=[0.5 0.5]  seed=724572  IsProcessed=on  isConnected=1
  Set Loss State : simeventsattributes2/Set Attribute  Priority=1  DialogController=des_ddg_create  DialogControllerArgs=DataTag81  SystemSampleTime=-1  AttributeFrom=Signal port  AttributeName=RndLoss  AttributeTreatAsVector=1  AttributeValue=1  AttributeCreate=on  StatNumberDeparted=Off  EvaluatedAttributeValue={[]}
  Signal Latch : simeventssignalmanage1/Signal Latch  Priority=1  SystemSampleTime=-1  InitialMemoryValue=0  WriteMemoryUpon=Trigger from port wtr  MemoryWriteEdgeOption=Rising  SpecifyWriteEventPriority=on  PriorityMemoryWrite=7000  ReadMemoryUpon=Trigger from port rtr  MemoryReadEdgeOption=Falling  SpecifyReadEventPriority=on  PriorityMemoryRead=200  ReportMemoryState=on  ReportMemoryUponWrite=off  ReportMemoryUponRead=off
  Signal Latch1 : simeventssignalmanage1/Signal Latch  Priority=1  SystemSampleTime=-1  InitialMemoryValue=1  WriteMemoryUpon=Sample time hit from port wts  MemoryWriteEdgeOption=Either  SpecifyWriteEventPriority=on  PriorityMemoryWrite=2200  ReadMemoryUpon=Write to memory event  MemoryReadEdgeOption=Falling  SpecifyReadEventPriority=on  PriorityMemoryRead=7000  ReportMemoryState=off  ReportMemoryUponWrite=off  ReportMemoryUponRead=on
  background4 : Subsystem
      mask Display: disp('')
  TX1 : PMIOPort  Port=1  Side=Left
  RX1 : PMIOPort  Port=2  Side=Left
  TX2 : PMIOPort  Port=3  Side=Left
  RX2 : PMIOPort  Port=4  Side=Left
  TX3 : PMIOPort  Port=5  Side=Left
  RX3 : PMIOPort  Port=6  Side=Left
  #p : Outport  OutDataType=sfix(16)  OutScaling=2^0
  util : Outport  Port=2  OutDataType=sfix(16)  OutScaling=2^0
  wires:
  Arbitration on Message Priority/3 -> util/1
  Arbitration on Message Priority/2 -> #p/1
  Arbitration on Message Priority/1 -> Signal Latch/2, Signal Latch/1
  Ground/1 -> Signal Latch/3
  Signal Latch/1 -> Flow Controller/1(Busy)
  RndLoss/1 -> Set Loss State/1
  Flow Controller/1(open) -> Signal Latch1/1, Signal Latch1/2
  Signal Latch1/1 -> Collision Detection/1
  connections:
  Arbitration on Message Priority/RConn2 -- Bounced Frames/LConn1
  Set Loss State/RConn1 -- Arbitration on Message Priority/LConn1
  Collision Detection/RConn1 -- Set Loss State/LConn1
  RX3/RConn1 -- Replicate/RConn3
  RX2/RConn1 -- Replicate/RConn2
  RX1/RConn1 -- Replicate/RConn1
  TX3/RConn1 -- Path Combiner/LConn3
  TX2/RConn1 -- Path Combiner/LConn2
  TX1/RConn1 -- Path Combiner/LConn1
  Arbitration on Message Priority/RConn1 -- Replicate/LConn1
  Path Combiner/RConn1 -- Collision Detection/LConn1
